simulink model "model_pompy"  (R2015a)
settings: Solver=ode4  StartTime=0.0  StopTime=T_sim  FixedStep=0.05  RelTol=1e-3
values from neighbouring files (symbols this model uses):
  h0 = poziom(1)    [chka_pompy.m]    (also in skryptDoIdentyfikacji.m; wskaznikJakosci.m)
  p1 = polyfit(PWM_level, pred_napelniania, 2)    [chka_pompy.m]    (also in skryptDoIdentyfikacji.m = [-53.386904761904304 2.090089285714280e+02 -16.6282738095236; wskaznikJakosci.m = [-53.386904761904304 2.090089285714280e+02 -16.6282738095236)
  PWM = 0.3    [chka_pompy.m]    (also in skryptDoIdentyfikacji.m = 0.9; wskaznikJakosci.m = 0.9)
  tau1 = tauP1(1) * PWM^3 + tauP1(2) * PWM^2 + tauP1(3) * PWM + tauP1(4)    [chka_pompy.m]
settings Model: Creator=konra  LastModifiedBy=konra
settings DataIOCC: LimitDataPoints=off

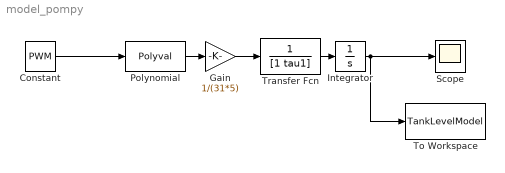
== system model_pompy ==
  Constant : Constant  Value=PWM
  Gain : Gain  Gain=1/(31*5)
  Integrator : Integrator  InitialCondition=h0
  Polynomial : Polyval  Coefs=p1
  Scope : Scope
  To Workspace : ToWorkspace  VariableName=TankLevelModel  SaveFormat=Structure With Time  SampleTime=-1
  Transfer Fcn : TransferFcn  Denominator=[1 tau1]
  wires:
  Gain/1 -> Transfer Fcn/1
  Integrator/1 -> To Workspace/1, Scope/1
  Constant/1 -> Polynomial/1
  Polynomial/1 -> Gain/1
  Transfer Fcn/1 -> Integrator/1
